simulink model "observer"  (R2024b)
settings: Solver=VariableStepAuto  StartTime=0.0  StopTime=10.0  RelTol=1e-3
values from neighbouring files (symbols this model uses):
  A = [0, -1 ... (first row only)    [d3.m]
  B = [1 ... (first row only)    [d3.m]
  C = [1, 0]    [d3.m]
  D = 0    [d3.m]
  K = acker(A,B, p_reg)    [d3.m]
  kr = 1 / dcgain(Wsp0)    [d3.m]
  L = acker(A', C', p_est)'    [d3.m]
  r = 10    [d3.m]
  x0 = [3 ... (first row only)    [d3.m]
settings Model: Creator=Korisnik  LastModifiedBy=Korisnik

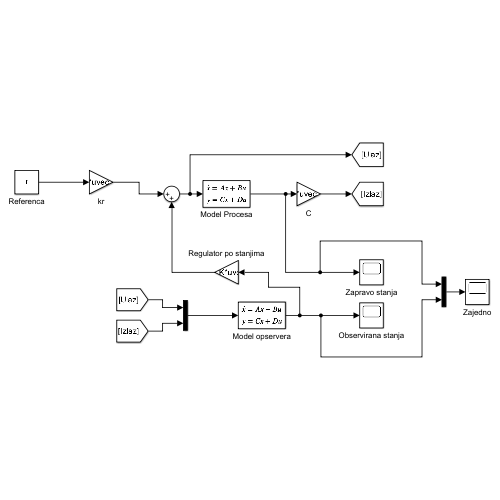
[thumbnail: Simulink's stored preview of the top-level diagram]
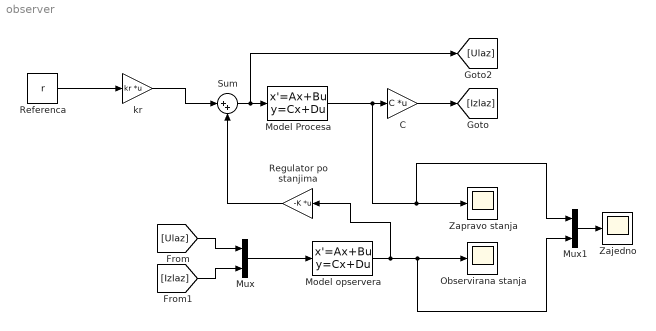
== system observer ==
  C : Gain  Gain=C  Multiplication=Matrix(K*u) (u vector)
  Model Procesa : StateSpace  A=A  B=B  C=[C; 0, 1]  D=[D; 0]  InitialCondition=x0
  Model opservera : StateSpace  A=A - L.*C  B=[B, L]  C=eye(2)  D=zeros(2)  InitialCondition=zeros(2,1)
  Mux : Mux  Inputs=2
  Mux1 : Mux  Inputs=2
  Observirana stanja : Scope
  Referenca : Constant  Value=r
  Regulator po stanjima : Gain  Gain=-K  Multiplication=Matrix(K*u) (u vector)
  Sum : Sum  Inputs=|++
  Zajedno : Scope
  Zapravo stanja : Scope
  kr : Gain  Gain=kr  Multiplication=Matrix(K*u) (u vector)
  wires:
  Model Procesa/1 -> Mux1/1, Zapravo stanja/1, C/1
  C/1 -> [Izlaz]
  [Izlaz] -> Mux/2
  [Ulaz] -> Mux/1
  Mux/1 -> Model opservera/1
  Model opservera/1 -> Regulator po stanjima/1, Mux1/2, Observirana stanja/1
  Mux1/1 -> Zajedno/1
  Sum/1 -> [Ulaz], Model Procesa/1
  Regulator po stanjima/1 -> Sum/2
  Referenca/1 -> kr/1
  kr/1 -> Sum/1
